simulink library "command_generation"  (R2016b)
settings: Solver=VariableStepAuto  StartTime=0.0  StopTime=10.0  RelTol=1e-3
libraries: momentum_dump_lib x1, command_processing x1
settings Model: Creator=taylorreynolds  LastModifiedBy=Taylor

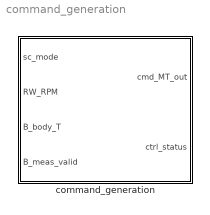
== system command_generation ==
  command_generation : Subsystem

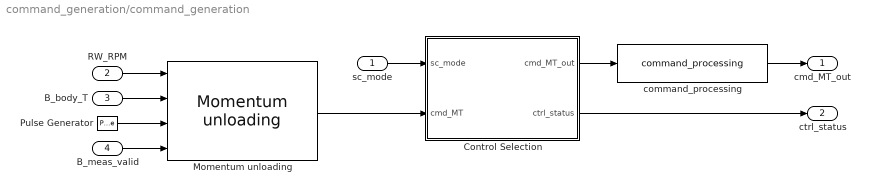
== system command_generation/command_generation ==
  sc_mode : Inport
  RW_RPM : Inport  Port=2
  B_body_T : Inport  Port=3
  B_meas_valid : Inport  Port=4
  Control Selection : Subsystem
  Momentum unloading : momentum_dump_lib/Momentum unloading
  Pulse Generator : DiscretePulseGenerator  PulseType=Time based  Period=fsw_params.actuators.ppt.sync_pulse  PulseWidth=fsw_params.actuators.ppt.t_charge_pct
  command_processing : command_processing/command_processing
  cmd_MT_out : Outport
  ctrl_status : Outport  Port=2
  wires:
  RW_RPM/1 -> Momentum unloading/1
  B_body_T/1 -> Momentum unloading/2
  Pulse Generator/1 -> Momentum unloading/3
  B_meas_valid/1 -> Momentum unloading/4
  command_processing/1 -> cmd_MT_out/1
  Control Selection/1("cmd_MT_out ") -> command_processing/1
  Control Selection/2(ctrl_status) -> ctrl_status/1
  sc_mode/1 -> Control Selection/1(sc_mode)
  Momentum unloading/1 -> Control Selection/2(cmd_MT)

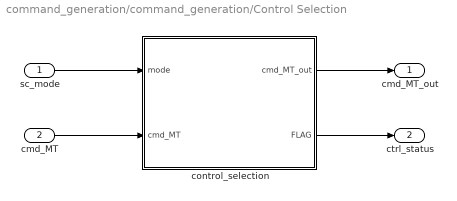
== system command_generation/command_generation/Control Selection ==
  sc_mode : Inport
  cmd_MT : Inport  Port=2
  control_selection : MATLAB Function  TreatAsAtomicUnit=on
  "cmd_MT_out " : Outport
  ctrl_status : Outport  Port=2
  wires:
  sc_mode/1 -> control_selection/1(mode)
  cmd_MT/1 -> control_selection/2(cmd_MT)
  control_selection/1(cmd_MT_out) -> "cmd_MT_out "/1
  control_selection/2(FLAG) -> ctrl_status/1

== matlab function command_generation/Control Selection/control_selection ==
  data: mode input; cmd_MT input; cmd_MT_out output; FLAG output
 function [cmd_MT_out,FLAG] = control_selection(mode,cmd_MT)
% Control Selection Logic
%   HuskySat-1, ADCS Team
%   Last Update: T. Reynolds, 11.21.17

% Selects which command gets passed to the actuators based on the mode
% provided by upstream mode selection. Current modes are:
%   mode_logic.bdot             = 1;
%   mode_logic.desat_eclipse    = 2;
%   mode_logic.point            = 3;
%       point.velocity          = 31;
%       point.ground            = 32;
%       point.MPC               = 33;
%   mode_logic.low_power        = 4;
%
% FLAG output can be used to make sure the control output matches up with
% what is being commanded, before commands are passed to actuators. FLAG
% should match mode, unless something is wrong.

FLAG    = 1;

if mode == 1 
    cmd_MT_out      = zeros(3,1);
elseif mode == 2
    cmd_MT_out      = cmd_MT;
elseif( mode == 31 || mode == 32 || mode == 33 )
    cmd_MT_out      = cmd_MT;
elseif mode == 4
    cmd_MT_out      = zeros(3,1);
else
    FLAG = -1;
    cmd_MT_out      = zeros(3,1);
end
